simulink library "groundpass_predict_lib"  (R2018b)
settings: Solver=VariableStepAuto  StartTime=0.0  StopTime=10.0  RelTol=1e-3
undefined symbols (not defined in the file or in its folder): Earth, fswParams, WGS84
libraries: aerolibtransform2 x4, vrlib x2
settings Model: Creator=colem  LastModifiedBy=colem

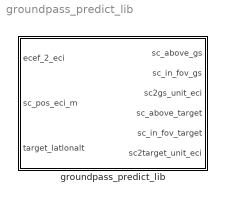
== system groundpass_predict_lib ==
  groundpass_predict_lib : Subsystem

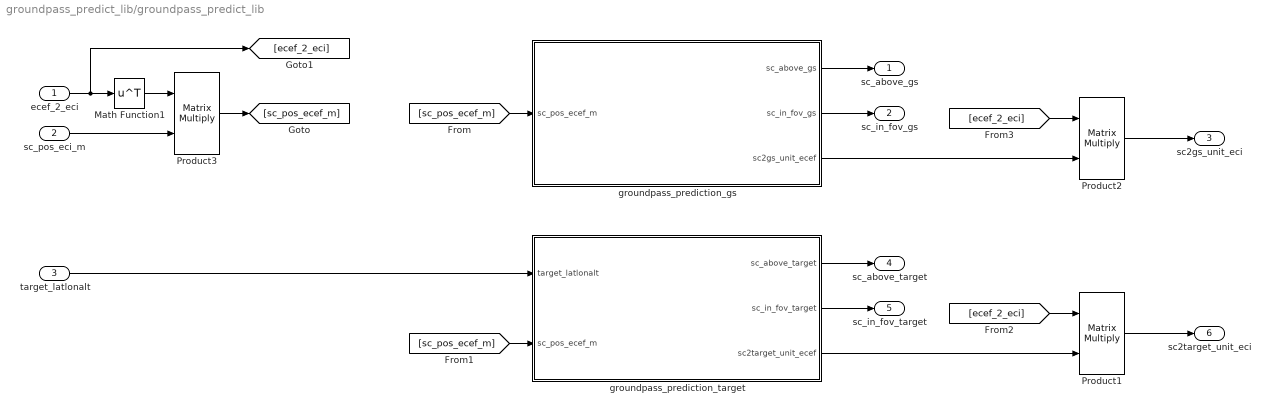
== system groundpass_predict_lib/groundpass_predict_lib ==
  ecef_2_eci : Inport
  sc_pos_eci_m : Inport  Port=2
  target_latlonalt : Inport  Port=3
  Math Function1 : Math  Operator=transpose  SaturateOnIntegerOverflow=on
  Product1 : Product  Multiplication=Matrix(*)
  Product2 : Product  Multiplication=Matrix(*)
  Product3 : Product  Multiplication=Matrix(*)
  groundpass_prediction_gs : Subsystem
  groundpass_prediction_target : Subsystem
  sc_above_gs : Outport
  sc_in_fov_gs : Outport  Port=2
  sc2gs_unit_eci : Outport  Port=3
  sc_above_target : Outport  Port=4
  sc_in_fov_target : Outport  Port=5
  sc2target_unit_eci : Outport  Port=6
  wires:
  Product3/1 -> [sc_pos_ecef_m]
  ecef_2_eci/1 -> [ecef_2_eci], Math Function1/1
  Math Function1/1 -> Product3/1
  groundpass_prediction_gs/2(sc_in_fov_gs) -> sc_in_fov_gs/1
  groundpass_prediction_gs/1(sc_above_gs) -> sc_above_gs/1
  sc_pos_eci_m/1 -> Product3/2
  [sc_pos_ecef_m] -> groundpass_prediction_gs/1(sc_pos_ecef_m)
  [sc_pos_ecef_m] -> groundpass_prediction_target/2(sc_pos_ecef_m)
  target_latlonalt/1 -> groundpass_prediction_target/1(target_latlonalt)
  groundpass_prediction_target/2(sc_in_fov_target) -> sc_in_fov_target/1
  groundpass_prediction_target/1(sc_above_target) -> sc_above_target/1
  groundpass_prediction_target/3(sc2target_unit_ecef) -> Product1/2
  [ecef_2_eci] -> Product1/1
  Product1/1 -> sc2target_unit_eci/1
  groundpass_prediction_gs/3(sc2gs_unit_ecef) -> Product2/2
  [ecef_2_eci] -> Product2/1
  Product2/1 -> sc2gs_unit_eci/1

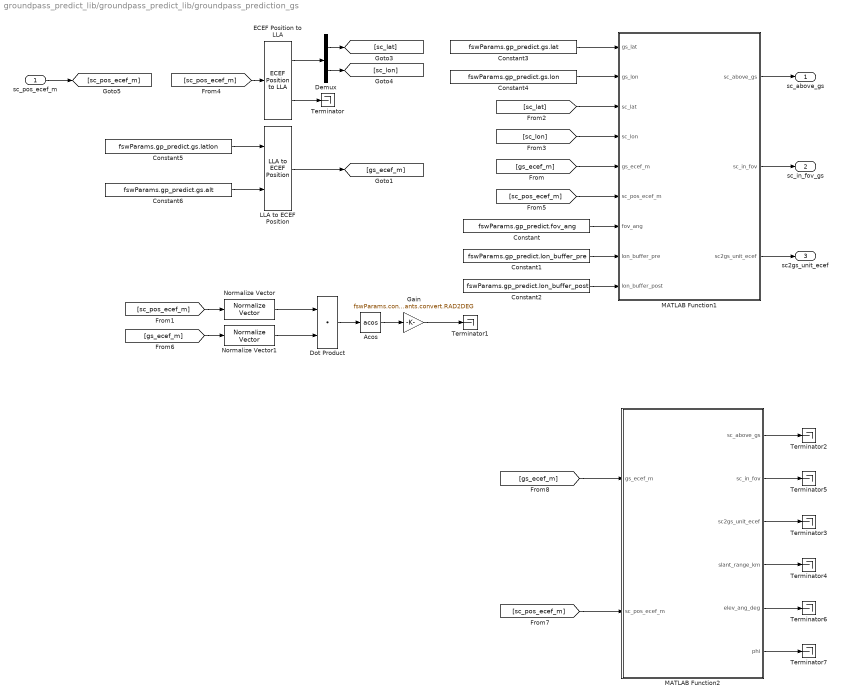
== system groundpass_predict_lib/groundpass_predict_lib/groundpass_prediction_gs ==
  sc_pos_ecef_m : Inport
  Acos : Trigonometry  Operator=acos
  Constant : Constant  Value=fswParams.gp_predict.fov_ang  SampleTime=fswParams.sample_time_s
  Constant1 : Constant  Value=fswParams.gp_predict.lon_buffer_pre  SampleTime=fswParams.sample_time_s
  Constant2 : Constant  Value=fswParams.gp_predict.lon_buffer_post  SampleTime=fswParams.sample_time_s
  Constant3 : Constant  Value=fswParams.gp_predict.gs.lat  SampleTime=fswParams.sample_time_s
  Constant4 : Constant  Value=fswParams.gp_predict.gs.lon  SampleTime=fswParams.sample_time_s
  Constant5 : Constant  Value=fswParams.gp_predict.gs.latlon  SampleTime=fswParams.sample_time_s
  Constant6 : Constant  Value=fswParams.gp_predict.gs.alt  SampleTime=fswParams.sample_time_s
  Demux : Demux  Outputs=[1 1]
  Dot Product : DotProduct  InputSameDT=on  OutDataTypeStr=Inherit: Inherit via internal rule
  ECEF Position to LLA : aerolibtransform2/ECEF Position to LLA  units=Metric (MKS)  ptype=Earth (WGS84)  F=1/298.257223563  R=6378137
      settings: SourceProductName=Aerospace Blockset  SourceProductBaseCode=AE
  Gain : Gain  Gain=fswParams.constants.convert.RAD2DEG
  LLA to ECEF Position : aerolibtransform2/LLA to ECEF Position  units=Metric (MKS)  ptype=Earth (WGS84)  F=1/298.257223563  R=6378137
      settings: SourceProductName=Aerospace Blockset  SourceProductBaseCode=AE
  MATLAB Function1 : MATLAB Function  TreatAsAtomicUnit=on
  MATLAB Function2 : MATLAB Function  TreatAsAtomicUnit=on
  Normalize Vector : vrlib/Utilities/Normalize Vector  maxzero=0
      settings: SourceProductName=Simulink 3D Animation  SourceProductBaseCode=VR
  Normalize Vector1 : vrlib/Utilities/Normalize Vector  maxzero=0
      settings: SourceProductName=Simulink 3D Animation  SourceProductBaseCode=VR
  Terminator{,1..7} (8 alike) : Terminator
  sc_above_gs : Outport
  sc_in_fov_gs : Outport  Port=2
  sc2gs_unit_ecef : Outport  Port=3
  wires:
  Constant/1 -> MATLAB Function1/7(fov_ang)
  MATLAB Function1/2(sc_in_fov) -> sc_in_fov_gs/1
  MATLAB Function1/3(sc2gs_unit_ecef) -> sc2gs_unit_ecef/1
  MATLAB Function1/1(sc_above_gs) -> sc_above_gs/1
  Constant3/1 -> MATLAB Function1/1(gs_lat)
  Constant4/1 -> MATLAB Function1/2(gs_lon)
  ECEF Position to LLA/2 -> Terminator/1
  Demux/1 -> [sc_lat]
  Demux/2 -> [sc_lon]
  ECEF Position to LLA/1 -> Demux/1
  [sc_lat] -> MATLAB Function1/3(sc_lat)
  [sc_lon] -> MATLAB Function1/4(sc_lon)
  sc_pos_ecef_m/1 -> [sc_pos_ecef_m]
  [sc_pos_ecef_m] -> ECEF Position to LLA/1
  [sc_pos_ecef_m] -> MATLAB Function1/6(sc_pos_ecef_m)
  [gs_ecef_m] -> MATLAB Function1/5(gs_ecef_m)
  Constant1/1 -> MATLAB Function1/8(lon_buffer_pre)
  Constant2/1 -> MATLAB Function1/9(lon_buffer_post)
  Constant5/1 -> LLA to ECEF Position/1
  Constant6/1 -> LLA to ECEF Position/2
  LLA to ECEF Position/1 -> [gs_ecef_m]
  [sc_pos_ecef_m] -> Normalize Vector/1
  [gs_ecef_m] -> Normalize Vector1/1
  Normalize Vector/1 -> Dot Product/1
  Normalize Vector1/1 -> Dot Product/2
  Dot Product/1 -> Acos/1
  Acos/1 -> Gain/1
  Gain/1 -> Terminator1/1
  [gs_ecef_m] -> MATLAB Function2/1(gs_ecef_m)
  [sc_pos_ecef_m] -> MATLAB Function2/2(sc_pos_ecef_m)
  MATLAB Function2/1(sc_above_gs) -> Terminator2/1
  MATLAB Function2/2(sc_in_fov) -> Terminator5/1
  MATLAB Function2/3(sc2gs_unit_ecef) -> Terminator3/1
  MATLAB Function2/4(slant_range_km) -> Terminator4/1
  MATLAB Function2/5(elev_ang_deg) -> Terminator6/1
  MATLAB Function2/6(phi) -> Terminator7/1

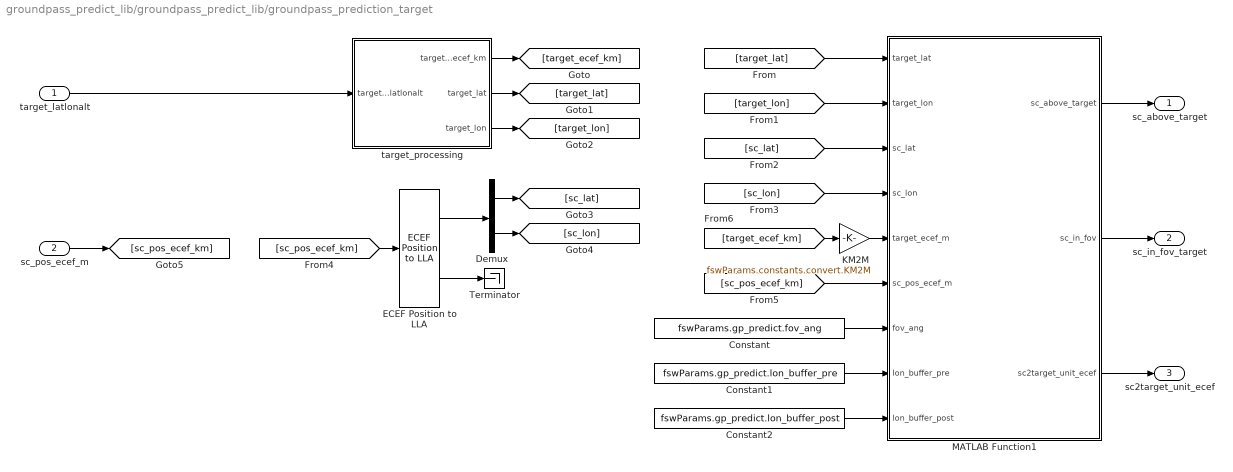
== system groundpass_predict_lib/groundpass_predict_lib/groundpass_prediction_target ==
  target_latlonalt : Inport
  sc_pos_ecef_m : Inport  Port=2
  Constant : Constant  Value=fswParams.gp_predict.fov_ang  SampleTime=fswParams.sample_time_s
  Constant1 : Constant  Value=fswParams.gp_predict.lon_buffer_pre  SampleTime=fswParams.sample_time_s
  Constant2 : Constant  Value=fswParams.gp_predict.lon_buffer_post  SampleTime=fswParams.sample_time_s
  Demux : Demux  Outputs=[1 1]
  ECEF Position to LLA : aerolibtransform2/ECEF Position to LLA  units=Metric (MKS)  ptype=Earth (WGS84)  F=1/298.257223563  R=6378137
      settings: SourceProductName=Aerospace Blockset  SourceProductBaseCode=AE
  KM2M : Gain  Gain=fswParams.constants.convert.KM2M
  MATLAB Function1 : MATLAB Function  TreatAsAtomicUnit=on
  Terminator : Terminator
  target_processing : Subsystem
  sc_above_target : Outport
  sc_in_fov_target : Outport  Port=2
  sc2target_unit_ecef : Outport  Port=3
  wires:
  Constant/1 -> MATLAB Function1/7(fov_ang)
  MATLAB Function1/2(sc_in_fov) -> sc_in_fov_target/1
  MATLAB Function1/3(sc2target_unit_ecef) -> sc2target_unit_ecef/1
  MATLAB Function1/1(sc_above_target) -> sc_above_target/1
  target_latlonalt/1 -> target_processing/1(target_latlonalt)
  target_processing/1(target_ecef_km) -> [target_ecef_km]
  target_processing/2(target_lat) -> [target_lat]
  target_processing/3(target_lon) -> [target_lon]
  [target_lat] -> MATLAB Function1/1(target_lat)
  [target_lon] -> MATLAB Function1/2(target_lon)
  ECEF Position to LLA/2 -> Terminator/1
  Demux/1 -> [sc_lat]
  Demux/2 -> [sc_lon]
  ECEF Position to LLA/1 -> Demux/1
  [sc_lat] -> MATLAB Function1/3(sc_lat)
  [sc_lon] -> MATLAB Function1/4(sc_lon)
  sc_pos_ecef_m/1 -> [sc_pos_ecef_km]
  [sc_pos_ecef_km] -> ECEF Position to LLA/1
  [sc_pos_ecef_km] -> MATLAB Function1/6(sc_pos_ecef_m)
  [target_ecef_km] -> KM2M/1
  KM2M/1 -> MATLAB Function1/5(target_ecef_m)
  Constant1/1 -> MATLAB Function1/8(lon_buffer_pre)
  Constant2/1 -> MATLAB Function1/9(lon_buffer_post)

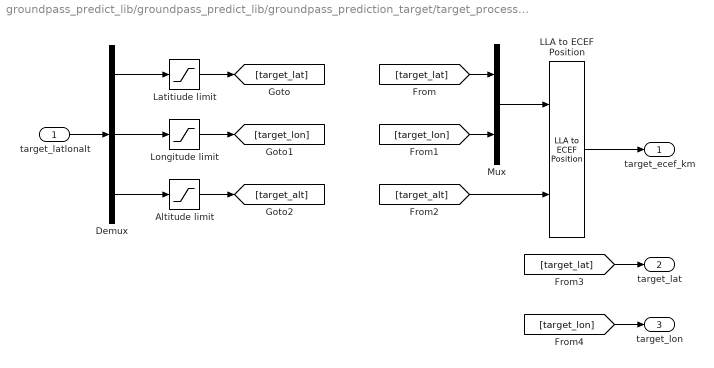
== system groundpass_predict_lib/groundpass_predict_lib/groundpass_prediction_target/target_processing ==
  target_latlonalt : Inport
  Altitude limit : Saturate  UpperLimit=inf  LowerLimit=0.01
  Demux : Demux  Outputs=[1 1 1]
  LLA to ECEF Position : aerolibtransform2/LLA to ECEF Position  units=Metric (MKS)  ptype=Earth (WGS84)  F=1/298.257223563  R=6378137
      settings: SourceProductName=Aerospace Blockset  SourceProductBaseCode=AE
  Latitiude limit : Saturate  UpperLimit=fswParams.gp_predict.target_lat_limit  LowerLimit=-fswParams.gp_predict.target_lat_limit
  Longitude limit : Saturate  UpperLimit=fswParams.gp_predict.target_lon_limit  LowerLimit=-fswParams.gp_predict.target_lon_limit
  Mux : Mux  Inputs=2
  target_ecef_km : Outport
  target_lat : Outport  Port=2
  target_lon : Outport  Port=3
  wires:
  Demux/2 -> Longitude limit/1
  Longitude limit/1 -> [target_lon]
  Demux/1 -> Latitiude limit/1
  LLA to ECEF Position/1 -> target_ecef_km/1
  Latitiude limit/1 -> [target_lat]
  Mux/1 -> LLA to ECEF Position/1
  Altitude limit/1 -> [target_alt]
  target_latlonalt/1 -> Demux/1
  Demux/3 -> Altitude limit/1
  [target_lat] -> Mux/1
  [target_lon] -> Mux/2
  [target_alt] -> LLA to ECEF Position/2
  [target_lat] -> target_lat/1
  [target_lon] -> target_lon/1

== matlab function groundpass_predict_lib/groundpass_prediction_gs/MATLAB Function2 ==
  data: gs_ecef_m input; sc_pos_ecef_m input; sc_above_gs output; sc_in_fov output; sc2gs_unit_ecef output; slant_range_km output; elev_ang_deg output; phi output
function [sc_above_gs,sc_in_fov,sc2gs_unit_ecef, slant_range_km, elev_ang_deg, phi] = ...
    sc_above_gs_elev(gs_ecef_m,sc_pos_ecef_m)



gs_vec         = gs_ecef_m;
sc_vec         = sc_pos_ecef_m;

gs_vec_unit    = gs_vec/norm(gs_vec);
sc_vec_unit    = sc_vec/norm(sc_vec);

slant_range_km = norm(gs_vec - sc_vec)/1000; 

%In ECEF coordinates
sc2gs_unit_ecef  = (gs_vec - sc_vec)/norm(gs_vec - sc_vec);

% Assume sc is not above gs.
sc_above_gs = 0;

% phi is the angle between the vector to the sc and the vector to the
% ground station. this is not the elevation angle, but it is one of the
% angles in the elevation angle triangle.
sin_phi = norm(cross(gs_vec, sc_vec))/(norm(gs_vec)*norm(sc_vec));
cos_phi = dot(gs_vec, sc_vec)/(norm(gs_vec)*norm(sc_vec));


phi     = atan2d(sin_phi, cos_phi); %degrees
    %also, if phi is < 90deg, the sc is on the correct side of earth
    
beta = asind(norm(gs_vec)*sind(phi)/norm(sc_vec - gs_vec)); 

% law of sines for this triangle.
% value minus 90 becuase elev angle is angle ABOVE horizon. 
% elev_ang_deg = -90 + asind(norm(sc_vec)*sind(phi)/norm(sc_vec - gs_vec));
elev_ang_deg = 180 - phi - beta - 90;

% Determine if the sc is above the horizon of the gs.
% Check if sc is within some elevation angle cone of the gs.

emin = 0.0 + 8.0;
emax = 180.0-emin;
if (elev_ang_deg > emin && elev_ang_deg < emax && phi < 90)
    sc_above_gs = 1;
end

% sc2gs_gs_dot  = dot(sc2gs_unit,gs_vec)/norm(gs_vec);
% 
% % Check LoS
% if sc2gs_gs_dot < 0
%     ABOVE     = TRUE;
% else
%     ABOVE     = FALSE;
% end
% 
% sc_above_gs = ABOVE;

pr = sc_vec - gs_vec;
fov_ang = 56/2;
fs = norm(pr)*cosd(fov_ang) - gs_vec'*pr/norm(gs_vec);
if (fs < 0)
    sc_in_fov = 1;
else
    sc_in_fov = 0;
end

== matlab function groundpass_predict_lib/groundpass_prediction_target/MATLAB Function1 ==
  data: target_lat input; target_lon input; sc_lat input; sc_lon input; target_ecef_m input; sc_above_target output; sc_in_fov output; sc2target_unit_ecef output; sc_pos_ecef_m input; fov_ang input; lon_buffer_pre input; lon_buffer_post input
function [sc_above_target,sc_in_fov,sc2target_unit_ecef] = ...
    sc_above_target(target_lat, target_lon, sc_lat, sc_lon, target_ecef_m,sc_pos_ecef_m,fov_ang,...
                                                                           lon_buffer_pre, lon_buffer_post)

% % Constants
% M2KM        = 1000;
% ECCE2       = 0.006694385000;
% RE          = 6378.137;
TRUE        = 1;
FALSE       = 0;
% -----

% Main Function

% Remnant from sun_vector, may not be relevant here?
% gs_eci_km(3)  = gs_eci_km(3)/(sqrt(1 - ECCE2));
% sc_pos_eci_km(3)        = sc_pos_eci_km(3)/(sqrt(1 - ECCE2));

target_vec     = target_ecef_m;
sc_vec         = sc_pos_ecef_m;

%In ECEF coordinates
sc2target_unit_ecef  = (target_vec - sc_vec)/norm(target_vec - sc_vec);

% Assume sc is not above target.
sc_above_target = false;

% Determine if the sc is above the horizon of the target.
% Check if sc lat lon is within some box around target lat lon
lat_check_1 = sc_lat < (target_lat + fov_ang);
lat_check_2 = sc_lat > (target_lat - fov_ang);
lon_check_1 = sc_lon > target_lon - lon_buffer_pre;
lon_check_2 = sc_lon < target_lon + lon_buffer_post;
if (lat_check_1 && lat_check_2 && lon_check_1 && lon_check_2  )
    sc_above_target = true;
end

% sc2target_target_dot  = dot(sc2target_unit,target_vec)/norm(target_vec);
% 
% % Check LoS
% if sc2target_target_dot < 0
%     ABOVE     = TRUE;
% else
%     ABOVE     = FALSE;
% end
% 
% sc_above_target = ABOVE;

pr = sc_vec - target_vec;
fs = norm(pr)*cosd(fov_ang) - target_vec'*pr/norm(target_vec);
if (fs < 0)
    sc_in_fov = true;
else
    sc_in_fov = false;
end

== matlab function groundpass_predict_lib/groundpass_prediction_gs/MATLAB Function1 ==
  data: gs_lat input; gs_lon input; sc_lat input; sc_lon input; gs_ecef_m input; sc_above_gs output; sc_in_fov output; sc2gs_unit_ecef output; sc_pos_ecef_m input; fov_ang input; lon_buffer_pre input; lon_buffer_post input
function [sc_above_gs,sc_in_fov,sc2gs_unit_ecef] = ...
    sc_above_gs(gs_lat, gs_lon, sc_lat, sc_lon, gs_ecef_m,sc_pos_ecef_m,fov_ang,...
                                                                           lon_buffer_pre, lon_buffer_post)

% % Constants
% M2KM        = 1000;
% ECCE2       = 0.006694385000;
% RE          = 6378.137;
TRUE        = 1;
FALSE       = 0;
% -----

% Main Function

% Remnant from sun_vector, may not be relevant here?
% gs_eci_km(3)  = gs_eci_km(3)/(sqrt(1 - ECCE2));
% sc_pos_eci_km(3)        = sc_pos_eci_km(3)/(sqrt(1 - ECCE2));

gs_vec         = gs_ecef_m;
sc_vec         = sc_pos_ecef_m;

%In ECEF coordinates
sc2gs_unit_ecef  = (gs_vec - sc_vec)/norm(gs_vec - sc_vec);

% Assume sc is not above gs.
sc_above_gs = false;

% Determine if the sc is above the horizon of the gs.
% Check if sc lat lon is within some box around gs lat lon
lat_check_1 = sc_lat < (gs_lat + fov_ang);
lat_check_2 = sc_lat > (gs_lat - fov_ang);
lon_check_1 = sc_lon > gs_lon - lon_buffer_pre;
lon_check_2 = sc_lon < gs_lon + lon_buffer_post;
if (lat_check_1 && lat_check_2 && lon_check_1 && lon_check_2  )
    sc_above_gs = true;
end

% sc2gs_gs_dot  = dot(sc2gs_unit,gs_vec)/norm(gs_vec);
% 
% % Check LoS
% if sc2gs_gs_dot < 0
%     ABOVE     = TRUE;
% else
%     ABOVE     = FALSE;
% end
% 
% sc_above_gs = ABOVE;

pr = sc_vec - gs_vec;
fs = norm(pr)*cosd(fov_ang) - gs_vec'*pr/norm(gs_vec);
if (fs < 0)
    sc_in_fov = true;
else
    sc_in_fov = false;
end
